simulink model "neuronchainv5"  (Simulink 7.6)
settings: Solver=ode45  StartTime=0.0  StopTime=200  RelTol=1e-3
values from neighbouring files (symbols this model uses):
  alpha = 0.8    [excneuroninit.m]
  beta = 0.05    [excneuroninit.m]
  inittime = 0.1    [excneuroninit.m]
  sensoryamp = 0.5    [excneuroninit.m]
  sigslopef = 1    [excneuroninit.m]
  sigslopei = 3    [excneuroninit.m]
  tau_s = 5    [excneuroninit.m]
libraries: simulink x500, neuronpoolibv3 x3
(part 18 of 18)

== system neuronchainv5/Subsystem/motoract vis inputs/Subsystem3 ==
  Saturation1 : Saturate  UpperLimit=1  LowerLimit=0
  Signal Generator2 : SignalGenerator  WaveForm=square
  Signal Generator3 : SignalGenerator  WaveForm=square  Frequency=0.5
  Sum1 : Sum  Inputs=|+-
  Tapped Delay{3..6} (4 alike) : simulink/Discrete/Tapped Delay  vinit=0.0  samptime=-1  NumDelays=1  DelayOrder=Oldest  includeCurrent=off
  Out1 : Outport
  Out2 : Outport  Port=2
  wires:
  Signal Generator2/1 -> Sum1/1
  Signal Generator3/1 -> Sum1/2
  Sum1/1 -> Saturation1/1
  Saturation1/1 -> Tapped Delay3/1, Out1/1
  Tapped Delay4/1 -> Tapped Delay5/1
  Tapped Delay3/1 -> Tapped Delay4/1
  Tapped Delay5/1 -> Tapped Delay6/1
  Tapped Delay6/1 -> Out2/1

== system neuronchainv5/Subsystem/motoract vis inputs/Subsystem4 ==
  Saturation1 : Saturate  UpperLimit=1  LowerLimit=0
  Signal Generator2 : SignalGenerator  WaveForm=square
  Signal Generator3 : SignalGenerator  WaveForm=square  Frequency=0.5
  Sum1 : Sum  Inputs=|+-
  Tapped Delay{3..6} (4 alike) : simulink/Discrete/Tapped Delay  vinit=0.0  samptime=-1  NumDelays=1  DelayOrder=Oldest  includeCurrent=off
  Out1 : Outport
  Out2 : Outport  Port=2
  wires:
  Signal Generator2/1 -> Sum1/1
  Signal Generator3/1 -> Sum1/2
  Sum1/1 -> Saturation1/1
  Saturation1/1 -> Tapped Delay3/1, Out1/1
  Tapped Delay4/1 -> Tapped Delay5/1
  Tapped Delay3/1 -> Tapped Delay4/1
  Tapped Delay5/1 -> Tapped Delay6/1
  Tapped Delay6/1 -> Out2/1
